simulink model "FIS_LQR_v01"  (R2024b)
settings: Solver=ode45  StartTime=0.0  StopTime=10  FixedStep=Ts  RelTol=1e-3
libraries: simulink x1, fuzblock x1
settings Model: Creator=ababaei  LastModifiedBy=ababaei
settings SolverCC: AlgebraicLoopSolver=LineSearch
settings DataIOCC: ExternalInput=[spg.setpoint.t, dist.Fz_IH]
settings DebuggingCC: AlgebraicLoopMsg=error  ArtificialAlgebraicLoopMsg=none  UnconnectedInputMsg=warning  UnconnectedOutputMsg=warning  UnconnectedLineMsg=warning  ArithmeticOperatorsInVariantConditions=warning
settings ModelReferenceCC: EnableRefExpFcnMdlSchedulingChecks=on
settings SFSimCC: SimUseLocalCustomCode=off  CustomCodeUndefinedFunction=UseInterfaceOnly
settings RTWCC: RTWUseLocalCustomCode=off  GPUComputeCapability=3.5
settings CodeAppCC: StateflowObjectComments=on

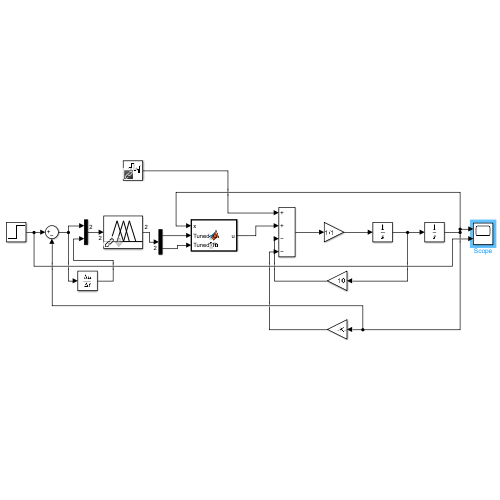
[thumbnail: Simulink's stored preview of the top-level diagram]
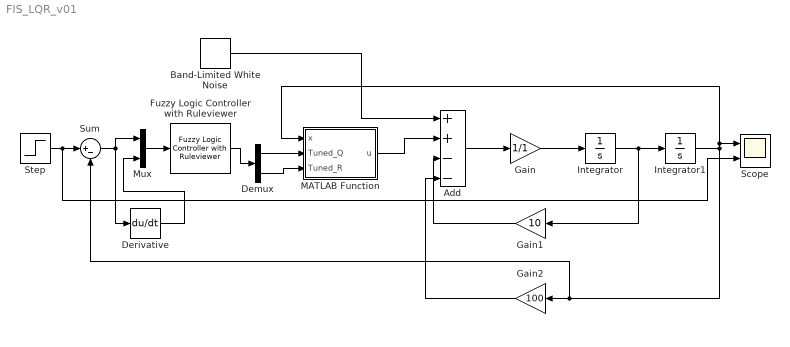
== system FIS_LQR_v01 ==
  Add : Sum  Inputs=++--
  Band-Limited White Noise : simulink/Sources/Band-Limited White Noise  Cov=[0.1]  Ts=0.1  seed=[23341]
  Demux : Demux  Outputs=2
  Derivative : Derivative
  Fuzzy Logic Controller with Ruleviewer : fuzblock/Fuzzy Logic  Controller  with Ruleviewer  fismatrix=mamdanitype1  Ts=2
  Gain : Gain  Gain=1/1
  Gain1 : Gain  Gain=10
  Gain2 : Gain  Gain=100
  Integrator : Integrator
  Integrator1 : Integrator
  MATLAB Function : MATLAB Function  TreatAsAtomicUnit=on
  Mux : Mux  Inputs=2
  Scope : Scope  NumInputPorts=2
  Step : Step  After=0  SampleTime=0
  Sum : Sum  Inputs=|+-
  wires:
  Integrator1/1 -> MATLAB Function/1(x), Scope/1, Gain2/1, Sum/2
  Integrator/1 -> Gain1/1, Integrator1/1
  Gain/1 -> Integrator/1
  Add/1 -> Gain/1
  Gain2/1 -> Add/4
  Gain1/1 -> Add/3
  Step/1 -> Scope/2, Sum/1
  MATLAB Function/1(u) -> Add/2
  Fuzzy Logic Controller with Ruleviewer/1 -> Demux/1
  Demux/1 -> MATLAB Function/2(Tuned_Q)
  Demux/2 -> MATLAB Function/3(Tuned_R)
  Mux/1 -> Fuzzy Logic Controller with Ruleviewer/1
  Sum/1 -> Derivative/1, Mux/1
  Derivative/1 -> Mux/2
  Band-Limited White Noise/1 -> Add/1

== matlab function FIS_LQR_v01/MATLAB Function ==
  data: x input; u output; Tuned_Q input; Tuned_R input
function u = fcn(x, Tuned_Q, Tuned_R)
    % Allow lqr to run outside the block
    coder.extrinsic('lqr');
    
    % Plant parameters
    A = [0 1; -100 -10];
    B = [0; 1];
    
    % Adaptive weighting matrices
    Q = [Tuned_Q 0; 0 Tuned_Q]; 
    R = Tuned_R;
    
    % Pre-define K and u to fix variable-size errors
    K = zeros(1, 2);
    u_raw = 0;
    
    % Compute optimal gain
    K = lqr(A, B, Q, R);
    
    % Compute control law and force scalar output
    u_raw = -K * x(:);
    u = double(u_raw(1)); 
end
%% Above is LQR which is a regulator controller for 0 input reference tracking 
% for non-zero tracking use below
% function u = fcn(x, Tuned_Q, Tuned_R, ref)
%     % Allow extrinsic calls for LQR calculation
%     coder.extrinsic('lqr');
% 
%     % Plant parameters (m=1, c=10, k=100)
%     A = [0 1; -100 -10];
%     B = [0; 1];
%     C = [1 0]; % Output is position
% 
%     % Adaptive weighting matrices
%     Q = [Tuned_Q 0; 0 Tuned_Q]; 
%     R = Tuned_R;
% 
%     % Initialize variables for code generation
%     K = zeros(1, 2);
%     u_raw = 0;
% 
%     % 1. Solve for optimal feedback gain K
%     K = lqr(A, B, Q, R);
% 
%     % 2. Calculate feedforward gain N for tracking
%     % Formula: N = -inv(C * inv(A - B*K) * B)
%     N = -1 / (C * ((A - B*K) \ B));
% 
%     % 3. Compute control law: u = -Kx + N*ref
%     u_raw = -K * x(:) + N * ref;
%     u = double(u_raw(1)); 
% end
%
